simulink model "v22_transmit"  (R2022a)
settings: Solver=FixedStepDiscrete  StartTime=0.0  StopTime=1  FixedStep=0.0016666666666666668  RelTol=1e-3
model workspace (MAT data in the model file):
  bps = 4
  fc = 1200
  frameBits = [0 1 1 1 1 1 1 0]
  inQ = [1+1i 3+1i 1+3i 3+3i]
  postamble = 120
  preamble = 300
  quadRot = [90 0 180 270]
  rrc = [0.00166950465783 0.00161541487245 0.00136077286171 0.000921868848776 0.000337964268746 -0.000331804375381 -0.00101405242267 -0.00162882202094 -0.00209855676539 -0.00235742969687 -0.00235997448449 -0.00208797727745 ... (129 elements, 1x129)]
  scrTaps = [14 17]
  syncBits = [1 1 1 1 1 1 1 0 0 0 0 1 1 1 0 1 1 1 1 0 0 1 0 1 1 0 0 1 0 0 1 0 0 0 0 0 0 1 0 0 0 1 0 0 1 1 0 0 0 1 0 1 1 1 0 1 0 1 1 0 1 1 0 0 0 0 0 1 1 0 0 1 1 0 1 0 1 0 0 1 1 1 0 0 1 1 1 1 0 1 1 0 1 0 0 0 0 1 0 1 0 1 0 1 1 1 1 1 0 1 0 0 1 0 1 0 0 0 1 1 0 1 1 1 0 0 0]
  syncGuard = 17
  syncLength = 127
settings Model: Creator=luoch  LastModifiedBy=luoch
settings DataIOCC: SaveOutput=off  SignalLogging=off
settings ModelReferenceCC: EnableRefExpFcnMdlSchedulingChecks=off
settings RTWCC: Description=Generic Real-Time Target  GPUComputeCapability=5.0
settings ConfigComp: CovBoundaryAbsTol=1.0e-5

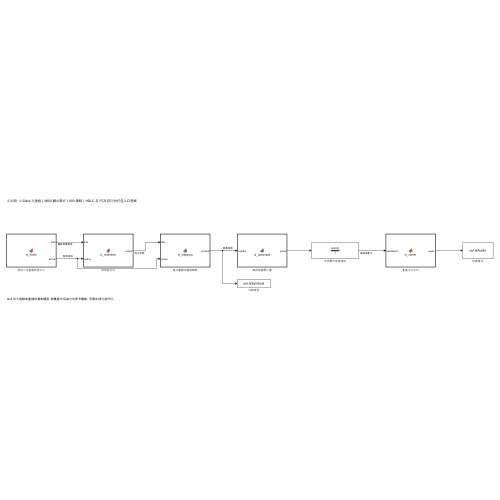
[thumbnail: Simulink's stored preview of the top-level diagram]
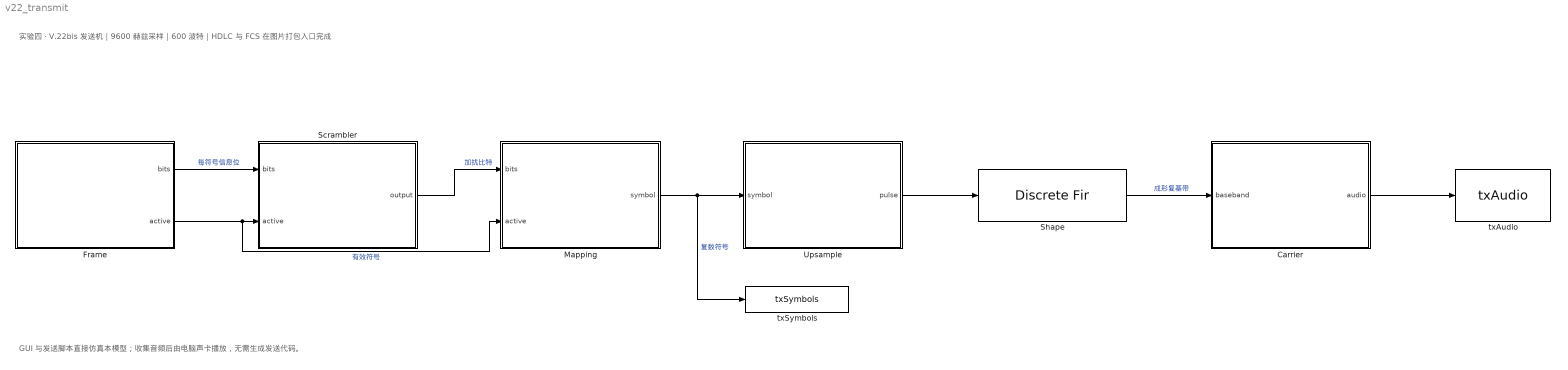
== system v22_transmit ==
  note: 实验四 · V.22bis 发送机｜9600 赫兹采样｜600 波特｜HDLC 与 FCS 在图片打包入口完成
  note: GUI 与发送脚本直接仿真本模型；收集音频后由电脑声卡播放，无需生成发送代码。
  Carrier : MATLAB Function  TreatAsAtomicUnit=on
      settings: AttributesFormatString=复基带上变频
  Frame : MATLAB Function  TreatAsAtomicUnit=on
      settings: AttributesFormatString=前后导与首尾同步标记
  Mapping : MATLAB Function  TreatAsAtomicUnit=on
      settings: AttributesFormatString=差分象限与幅度映射
  Scrambler : MATLAB Function  TreatAsAtomicUnit=on
      settings: AttributesFormatString=自同步扰码
  Shape : DiscreteFir  Coefficients=rrc  InputProcessing=Columns as channels (frame based)
      settings: AttributesFormatString=平方根升余弦成形
  Upsample : MATLAB Function  TreatAsAtomicUnit=on
      settings: AttributesFormatString=每符号插零扩展
  txAudio : ToWorkspace  VariableName=txAudio  SampleTime=-1
      settings: AttributesFormatString=仿真音频
  txSymbols : ToWorkspace  VariableName=txSymbols  SampleTime=-1
      settings: AttributesFormatString=调制符号
  wires:
  Frame/1(bits) -> Scrambler/1(bits)  "每符号信息位"
  Frame/2(active) -> Scrambler/2(active), Mapping/2(active)  "有效符号"
  Scrambler/1(output) -> Mapping/1(bits)  "加扰比特"
  Mapping/1(symbol) -> Upsample/1(symbol), txSymbols/1  "复数符号"
  Upsample/1(pulse) -> Shape/1
  Shape/1 -> Carrier/1(baseband)  "成形复基带"
  Carrier/1(audio) -> txAudio/1

== matlab function v22_transmit/Scrambler ==
  settings: updateMethod=DISCRETE  sampleTime=0.0016666666666666668
  data: bits input; output output; active input; bps parameter; scrTaps parameter
function output=tx_scrambler(bits,active,bps, scrTaps)
%#codegen
% 自同步扰码：当前信息位异或第 14 与第 17 个历史输出。
persistent state
if isempty(state),state=false(1,17);end
output=zeros(4,1);
if ~active,return,end
for k=1:bps
 value=xor(bits(k)~=0,xor(state(scrTaps(1)),state(scrTaps(2))));
 output(k)=double(value);state=[value state(1:end-1)];
end
end

== matlab function v22_transmit/Frame ==
  settings: updateMethod=DISCRETE  sampleTime=0.0016666666666666668
  data: bits output; active output; frameBits parameter; bps parameter; preamble parameter; postamble parameter; syncBits parameter; syncGuard parameter; syncLength parameter
function [bits,active]=tx_frame(frameBits,bps,preamble,postamble,syncBits,syncGuard,syncLength)
%#codegen
% 已组装的 HDLC 比特外，加入前后导及用于实验测量的首尾 m 序列。
persistent symbolIndex
if isempty(symbolIndex),symbolIndex=0;end
nSync=syncLength;nFrame=numel(frameBits);pre=preamble*bps;
total=pre+2*nSync+2*syncGuard+nFrame+postamble*bps;
active=symbolIndex<ceil(total/bps);bits=zeros(4,1);
for k=1:bps
 index=symbolIndex*bps+k;value=1;
 if index>total,value=0;
 elseif index>pre
  index=index-pre;
  if index<=nSync,value=syncBits(index);
  elseif index<=nSync+syncGuard,value=1;
  elseif index<=nSync+syncGuard+nFrame,value=frameBits(index-nSync-syncGuard);
  elseif index<=nSync+2*syncGuard+nFrame,value=1;
  elseif index<=2*nSync+2*syncGuard+nFrame,value=syncBits(index-nSync-2*syncGuard-nFrame);
  end
 end
 bits(k)=value;
end
symbolIndex=symbolIndex+1;
end

== matlab function v22_transmit/Mapping ==
  settings: updateMethod=DISCRETE  sampleTime=0.0016666666666666668
  data: bits input; symbol output; active input; bps parameter; quadRot parameter; inQ parameter
function symbol=tx_mapping(bits,active,bps, quadRot, inQ)
%#codegen
% 前两位控制相对旋转；16-QAM 后两位选择象限内幅度。
persistent quadrant
if isempty(quadrant),quadrant=0;end
symbol=complex(0);
if ~active,return,end
hi=2*bits(1)+bits(2);quadrant=mod(quadrant+quadRot(hi+1),360);
lo=0;if bps==4,lo=2*bits(3)+bits(4);end
symbol=inQ(lo+1)*exp(1i*quadrant*pi/180);
end

== matlab function v22_transmit/Upsample ==
  settings: updateMethod=DISCRETE  sampleTime=0.0016666666666666668
  data: symbol input; pulse output
function pulse=tx_upsample(symbol)
%#codegen
% 每符号 16 个采样点。
pulse=complex(zeros(16,1));pulse(1)=symbol;
end

== matlab function v22_transmit/Carrier ==
  settings: updateMethod=DISCRETE  sampleTime=0.0016666666666666668
  data: baseband input; audio output; fc parameter
function audio=tx_carrier(baseband,fc)
%#codegen
% 复基带上变频为实通带音频，载波相位跨符号连续。
persistent sample
if isempty(sample),sample=0;end
audio=real(baseband.*exp(1i*2*pi*fc*(sample+(0:15)')/9600));sample=sample+16;
end
